simulink subsystem "ros_command"  (R2024a)
settings: Solver=VariableStepAuto  StartTime=0.0  StopTime=10.0  RelTol=1e-3
undefined symbols (not defined in the file): MPC, simulink
libraries: ros2lib x43
settings Model: Creator=lamarre  LastModifiedBy=nimai
settings DebuggingCC: UnconnectedInputMsg=warning  UnconnectedOutputMsg=warning  UnconnectedLineMsg=warning
settings ModelReferenceCC: EnableRefExpFcnMdlSchedulingChecks=on
settings RTWCC: GPUComputeCapability=3.5  DLArmComputeVersion=19.05

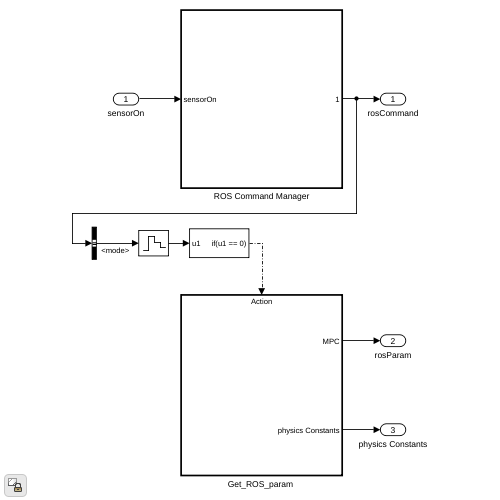
[thumbnail: Simulink's stored preview of the top-level diagram]
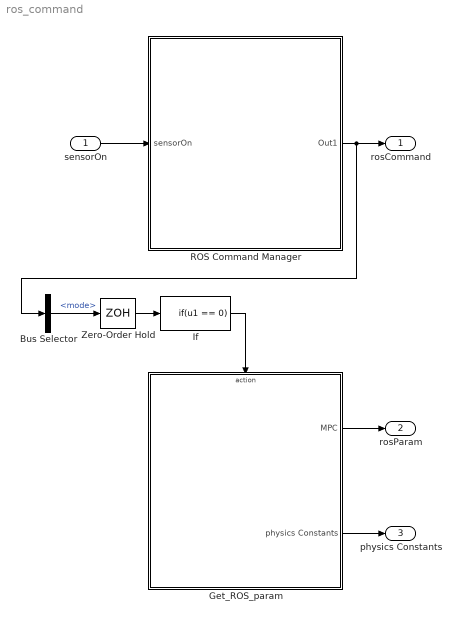
== system ros_command ==
  sensorOn : Inport
  Bus Selector : BusSelector  OutputSignals=mode
  "Get_ROS_param " : Subsystem
  If : If  IfExpression=u1 == 0  ShowElse=off
  ROS Command Manager : Subsystem  TreatAsAtomicUnit=on  SystemSampleTime=MPC.Ts
  Zero-Order Hold : ZeroOrderHold  SampleTime=simulink.ros.paramSampletime
  rosCommand : Outport
  rosParam : Outport  Port=2
  physics Constants : Outport  Port=3
  wires:
  sensorOn/1 -> ROS Command Manager/1(sensorOn)
  ROS Command Manager/1(Out1) -> Bus Selector/1, rosCommand/1
  If/1 -> "Get_ROS_param "/Action
  Bus Selector/1 -> Zero-Order Hold/1  "<mode>"
  "Get_ROS_param "/1(MPC) -> rosParam/1
  "Get_ROS_param "/2(physics Constants) -> physics Constants/1
  Zero-Order Hold/1 -> If/1

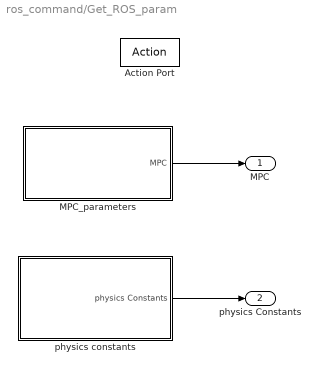
== system ros_command/Get_ROS_param  ==
  Action Port : ActionPort  InitializeStates=reset
  MPC_parameters : Subsystem
  physics constants : Subsystem
  MPC : Outport
  physics Constants : Outport  Port=2
  wires:
  physics constants/1(physics Constants) -> physics Constants/1
  MPC_parameters/1(MPC) -> MPC/1

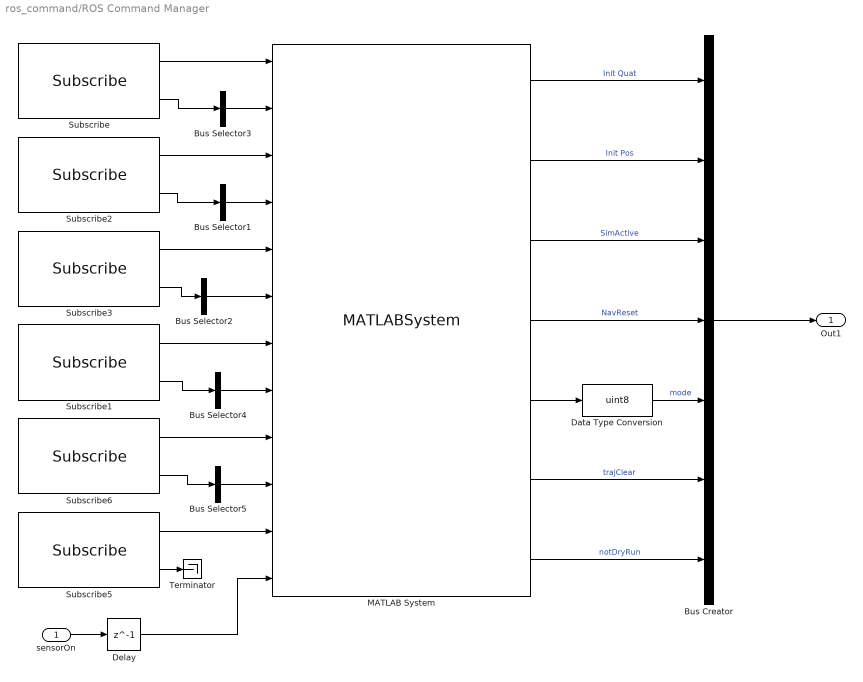
== system ros_command/ROS Command Manager ==
  sensorOn : Inport
  Bus Creator : BusCreator  Inputs=7
  Bus Selector{1..3,5} (4 alike) : BusSelector  OutputSignals=Data  OutputAsBus=on
  Bus Selector4 : BusSelector  OutputSignals=Position.X,Position.Y,Position.Z,Orientation.W,Orientation.X,Orientation.Y,Orientation.Z  OutputAsBus=on
  Data Type Conversion : DataTypeConversion  OutDataTypeStr=uint8  SaturateOnIntegerOverflow=off  RndMeth=Floor
  Delay : Delay  DelayLength=1  InitialCondition=0
  MATLAB System : MATLABSystem  System=rosCommandManager  initial_mode=mode.init  SimulateUsing=Code generation
      mask Type: rosCommandManager
      mask Display:
      | disp('rosCommandManager');
      | port_label('input',1,'newSetMode');
      | port_label('input',2,'setMode');
      | port_label('input',3,'newReset');
      | port_label('input',4,'reset');
      | port_label('input',5,'newKill');
      | port_label('input',6,'kill');
      | port_label('input',7,'newIc');
      | port_label('input',8,'ic');
      | port_label('input',9,'newDryRun');
      | port_label('input',10,'Dryrun');
      | port_label('input',11,'newTrajreset');
      | port_label('input',12,'sensorOn');
      | port_label('output',1,'initQuat');
      | port_label('output',2,'initPos');
      | port_label('output',3,'simEnable');
      | port_label('output',4,'reset');
      | port_label('output',5,'mode');
      | port_label('output',6,'trajClear');
      | port_label('output',7,'notDryRun');
  Subscribe : ros2lib/Subscribe  topicSource=Specify your own  topic=/proc_control/set_mode  messageType=std_msgs/UInt8  sampleTime=MPC.Ts  QOSHistory=Keep last  QOSDepth=1  QOSReliability=Reliable  QOSDurability=Volatile  QOSDeadline=Inf  QOSLifespan=Inf  QOSLiveliness=Automatic  QOSLeaseDuration=Inf  QOSAvoidROSNamespaceConventions=off
  Subscribe1 : ros2lib/Subscribe  topicSource=Specify your own  topic=/proc_simulation/start_simulation  messageType=geometry_msgs/Pose  sampleTime=MPC.Ts  QOSHistory=Keep last  QOSDepth=1  QOSReliability=Reliable  QOSDurability=Volatile  QOSDeadline=Inf  QOSLifespan=Inf  QOSLiveliness=Automatic  QOSLeaseDuration=Inf  QOSAvoidROSNamespaceConventions=off
  Subscribe2 : ros2lib/Subscribe  topicSource=Specify your own  topic=/proc_nav/reset_pos  messageType=std_msgs/Bool  sampleTime=MPC.Ts  QOSHistory=Keep last  QOSDepth=1  QOSReliability=Reliable  QOSDurability=Volatile  QOSDeadline=Inf  QOSLifespan=Inf  QOSLiveliness=Automatic  QOSLeaseDuration=Inf  QOSAvoidROSNamespaceConventions=off
  Subscribe3 : ros2lib/Subscribe  topicSource=Specify your own  topic=/provider_rs485/kill_status  messageType=sonia_common_ros2/KillStatus  sampleTime=MPC.Ts  QOSHistory=Keep last  QOSDepth=1  QOSReliability=Reliable  QOSDurability=Volatile  QOSDeadline=Inf  QOSLifespan=Inf  QOSLiveliness=Automatic  QOSLeaseDuration=Inf  QOSAvoidROSNamespaceConventions=off
  Subscribe5 : ros2lib/Subscribe  topicSource=Specify your own  topic=/proc_control/reset_trajectory  messageType=std_msgs/Bool  sampleTime=MPC.Ts  QOSHistory=Keep last  QOSDepth=1  QOSReliability=Reliable  QOSDurability=Volatile  QOSDeadline=Inf  QOSLifespan=Inf  QOSLiveliness=Automatic  QOSLeaseDuration=Inf  QOSAvoidROSNamespaceConventions=off
  Subscribe6 : ros2lib/Subscribe  topicSource=Specify your own  topic=/telemetry/dry_run  messageType=std_msgs/Bool  sampleTime=MPC.Ts  QOSHistory=Keep last  QOSDepth=1  QOSReliability=Reliable  QOSDurability=Volatile  QOSDeadline=Inf  QOSLifespan=Inf  QOSLiveliness=Automatic  QOSLeaseDuration=Inf  QOSAvoidROSNamespaceConventions=off
  Terminator : Terminator
  Out1 : Outport
  wires:
  Subscribe2/1 -> MATLAB System/3
  Bus Selector5/1 -> MATLAB System/10
  Subscribe1/2 -> Bus Selector4/1
  Subscribe/1 -> MATLAB System/1
  MATLAB System/4 -> Bus Creator/4  "NavReset"
  Subscribe5/1 -> MATLAB System/11
  Bus Selector2/1 -> MATLAB System/6
  Bus Creator/1 -> Out1/1
  Bus Selector4/1 -> MATLAB System/8
  Subscribe2/2 -> Bus Selector1/1
  MATLAB System/7 -> Bus Creator/7  "notDryRun"
  Data Type Conversion/1 -> Bus Creator/5  "mode"
  sensorOn/1 -> Delay/1
  Subscribe5/2 -> Terminator/1
  Bus Selector3/1 -> MATLAB System/2
  Subscribe1/1 -> MATLAB System/7
  MATLAB System/3 -> Bus Creator/3  "SimActive"
  Subscribe6/2 -> Bus Selector5/1
  Subscribe3/1 -> MATLAB System/5
  Subscribe/2 -> Bus Selector3/1
  Subscribe3/2 -> Bus Selector2/1
  Bus Selector1/1 -> MATLAB System/4
  Delay/1 -> MATLAB System/12
  Subscribe6/1 -> MATLAB System/9
  MATLAB System/6 -> Bus Creator/6  "trajClear"
  MATLAB System/2 -> Bus Creator/2  "Init Pos"
  MATLAB System/5 -> Data Type Conversion/1
  MATLAB System/1 -> Bus Creator/1  "Init Quat"

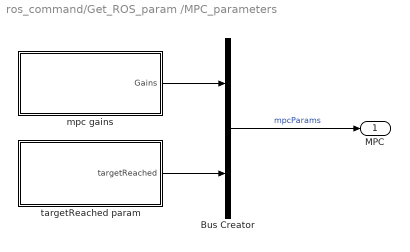
== system ros_command/Get_ROS_param /MPC_parameters ==
  Bus Creator : BusCreator  Inputs=2  OutDataTypeStr=Bus: mpcParams  NonVirtualBus=on
  mpc gains : Subsystem
  targetReached param : Subsystem
  MPC : Outport
  wires:
  Bus Creator/1 -> MPC/1  "mpcParams"
  mpc gains/1(Gains) -> Bus Creator/1
  targetReached param/1(targetReached) -> Bus Creator/2

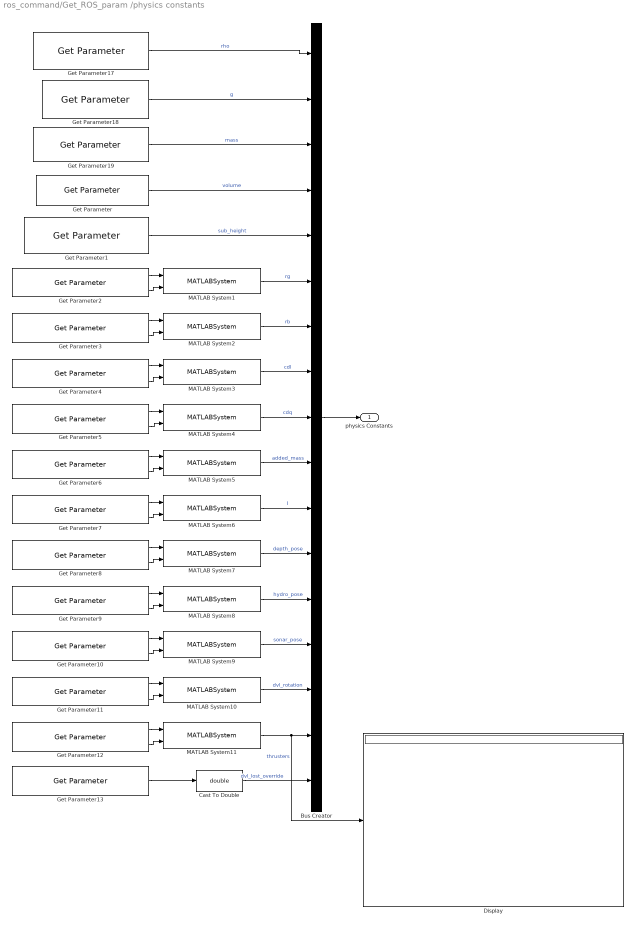
== system ros_command/Get_ROS_param /physics constants ==
  Bus Creator : BusCreator  Inputs=17  OutDataTypeStr=Bus: physicsConstants  NonVirtualBus=on
  Cast To Double : DataTypeConversion  OutDataTypeStr=double  SaturateOnIntegerOverflow=off  RndMeth=Floor
  Display : Display
  Get Parameter : ros2lib/Get Parameter  ParameterName=proc_control.physics.volume  ParameterType=double  ParameterMaxArrayLength=16  ParameterInitialValue=physics.volume  SampleTime=-1  ModelName=proc_control  BlockId=ParamGet_proc_control_185_615
  Get Parameter1 : ros2lib/Get Parameter  ParameterName=proc_control.physics.sub_height  ParameterType=double  ParameterMaxArrayLength=16  ParameterInitialValue=physics.height  SampleTime=-1  ModelName=proc_control  BlockId=ParamGet_proc_control_185_616
  Get Parameter10 : ros2lib/Get Parameter  ParameterName=proc_control.physics.sonar_pose  ParameterType=uint8[]  ParameterMaxArrayLength=64  ParameterInitialValue=int8('0,0,0')  SampleTime=-1  ModelName=proc_control  BlockId=ParamGet_proc_control_185_626
  Get Parameter11 : ros2lib/Get Parameter  ParameterName=proc_control.physics.dvl_rotation  ParameterType=uint8[]  ParameterMaxArrayLength=64  ParameterInitialValue=int8('0,0,0')  SampleTime=-1  ModelName=proc_control  BlockId=ParamGet_proc_control_185_627
  Get Parameter12 : ros2lib/Get Parameter  ParameterName=proc_control.physics.thrusters  ParameterType=uint8[]  ParameterMaxArrayLength=400  ParameterInitialValue=int8('0,0,0')  SampleTime=-1  ModelName=proc_control  BlockId=ParamGet_proc_control_185_628
  Get Parameter13 : ros2lib/Get Parameter  ParameterName=proc_control.physics.dvl_lost_override  ParameterType=boolean  ParameterMaxArrayLength=400  ParameterInitialValue=true  SampleTime=-1  ModelName=proc_control  BlockId=ParamGet_proc_control_185_629
  Get Parameter17 : ros2lib/Get Parameter  ParameterName=proc_control.physics.rho  ParameterType=double  ParameterMaxArrayLength=16  ParameterInitialValue=physics.rho  SampleTime=-1  ModelName=proc_control  BlockId=ParamGet_proc_control_185_612
  Get Parameter18 : ros2lib/Get Parameter  ParameterName=proc_control.physics.g  ParameterType=double  ParameterMaxArrayLength=16  ParameterInitialValue=physics.g  SampleTime=-1  ModelName=proc_control  BlockId=ParamGet_proc_control_185_613
  Get Parameter19 : ros2lib/Get Parameter  ParameterName=proc_control.physics.mass  ParameterType=double  ParameterMaxArrayLength=16  ParameterInitialValue=physics.mass  SampleTime=-1  ModelName=proc_control  BlockId=ParamGet_proc_control_185_614
  Get Parameter2 : ros2lib/Get Parameter  ParameterName=proc_control.physics.rg  ParameterType=uint8[]  ParameterMaxArrayLength=64  ParameterInitialValue=int8('0,0,0')  SampleTime=-1  ModelName=proc_control  BlockId=ParamGet_proc_control_185_617
  Get Parameter3 : ros2lib/Get Parameter  ParameterName=proc_control.physics.rb  ParameterType=uint8[]  ParameterMaxArrayLength=64  ParameterInitialValue=int8('0,0,0')  SampleTime=-1  ModelName=proc_control  BlockId=ParamGet_proc_control_185_618
  Get Parameter4 : ros2lib/Get Parameter  ParameterName=proc_control.physics.cdl  ParameterType=uint8[]  ParameterMaxArrayLength=64  ParameterInitialValue=int8('0,0,0,0,0,0')  SampleTime=-1  ModelName=proc_control  BlockId=ParamGet_proc_control_185_619
  Get Parameter5 : ros2lib/Get Parameter  ParameterName=proc_control.physics.cdq  ParameterType=uint8[]  ParameterMaxArrayLength=64  ParameterInitialValue=int8('0,0,0,0,0,0')  SampleTime=-1  ModelName=proc_control  BlockId=ParamGet_proc_control_185_620
  Get Parameter6 : ros2lib/Get Parameter  ParameterName=proc_control.physics.added_mass  ParameterType=uint8[]  ParameterMaxArrayLength=64  ParameterInitialValue=int8('0,0,0,0,0,0')  SampleTime=-1  ModelName=proc_control  BlockId=ParamGet_proc_control_185_621
  Get Parameter7 : ros2lib/Get Parameter  ParameterName=proc_control.physics.I  ParameterType=uint8[]  ParameterMaxArrayLength=128  ParameterInitialValue=int8('0,0,0,0,0,0,0,0,0')  SampleTime=-1  ModelName=proc_control  BlockId=ParamGet_proc_control_185_622
  Get Parameter8 : ros2lib/Get Parameter  ParameterName=proc_control.physics.depth_pose  ParameterType=uint8[]  ParameterMaxArrayLength=64  ParameterInitialValue=int8('0,0,0')  SampleTime=-1  ModelName=proc_control  BlockId=ParamGet_proc_control_185_623
  Get Parameter9 : ros2lib/Get Parameter  ParameterName=proc_control.physics.hydro_pose  ParameterType=uint8[]  ParameterMaxArrayLength=64  ParameterInitialValue=int8('0,0,0')  SampleTime=-1  ModelName=proc_control  BlockId=ParamGet_proc_control_185_625
  MATLAB System1 : MATLABSystem  System=String2DoubleArray  arraySize=[1, 3]  constantName='Center of Mass'  SimulateUsing=Code generation
      mask Type: String2DoubleArray
      mask Display:
      | disp('String2DoubleArray');
      | port_label('input',1,'string');
      | port_label('input',2,'length');
      | port_label('output',1,'array');
  MATLAB System10 : MATLABSystem  System=String2DoubleArray  arraySize=[1, 3]  constantName='DVL Rotation'  SimulateUsing=Code generation
      mask Type: String2DoubleArray
      mask Display:
      | disp('String2DoubleArray');
      | port_label('input',1,'string');
      | port_label('input',2,'length');
      | port_label('output',1,'array');
  MATLAB System11 : MATLABSystem  System=String2DoubleArray  arraySize=[MPC.nu 6]  constantName='Thrusters Config'  SimulateUsing=Code generation
      mask Type: String2DoubleArray
      mask Display:
      | disp('String2DoubleArray');
      | port_label('input',1,'string');
      | port_label('input',2,'length');
      | port_label('output',1,'array');
  MATLAB System2 : MATLABSystem  System=String2DoubleArray  arraySize=[1, 3]  constantName='Center of Buoyancy'  SimulateUsing=Code generation
      mask Type: String2DoubleArray
      mask Display:
      | disp('String2DoubleArray');
      | port_label('input',1,'string');
      | port_label('input',2,'length');
      | port_label('output',1,'array');
  MATLAB System3 : MATLABSystem  System=String2DoubleArray  arraySize=[1,6]  constantName='Linear drag constant'  SimulateUsing=Code generation
      mask Type: String2DoubleArray
      mask Display:
      | disp('String2DoubleArray');
      | port_label('input',1,'string');
      | port_label('input',2,'length');
      | port_label('output',1,'array');
  MATLAB System4 : MATLABSystem  System=String2DoubleArray  arraySize=[1, 6]  constantName='Quadratic drag constant'  SimulateUsing=Code generation
      mask Type: String2DoubleArray
      mask Display:
      | disp('String2DoubleArray');
      | port_label('input',1,'string');
      | port_label('input',2,'length');
      | port_label('output',1,'array');
  MATLAB System5 : MATLABSystem  System=String2DoubleArray  arraySize=[1, 6]  constantName='Added Mass'  SimulateUsing=Code generation
      mask Type: String2DoubleArray
      mask Display:
      | disp('String2DoubleArray');
      | port_label('input',1,'string');
      | port_label('input',2,'length');
      | port_label('output',1,'array');
  MATLAB System6 : MATLABSystem  System=String2DoubleArray  arraySize=[1,9]  constantName='Inertia Tensor'  SimulateUsing=Code generation
      mask Type: String2DoubleArray
      mask Display:
      | disp('String2DoubleArray');
      | port_label('input',1,'string');
      | port_label('input',2,'length');
      | port_label('output',1,'array');
  MATLAB System7 : MATLABSystem  System=String2DoubleArray  arraySize=[1, 3]  constantName='Depth Pose'  SimulateUsing=Code generation
      mask Type: String2DoubleArray
      mask Display:
      | disp('String2DoubleArray');
      | port_label('input',1,'string');
      | port_label('input',2,'length');
      | port_label('output',1,'array');
  MATLAB System8 : MATLABSystem  System=String2DoubleArray  arraySize=[1, 3]  constantName='Hydro Pose'  SimulateUsing=Code generation
      mask Type: String2DoubleArray
      mask Display:
      | disp('String2DoubleArray');
      | port_label('input',1,'string');
      | port_label('input',2,'length');
      | port_label('output',1,'array');
  MATLAB System9 : MATLABSystem  System=String2DoubleArray  arraySize=[1, 3]  constantName='Sonar Pose'  SimulateUsing=Code generation
      mask Type: String2DoubleArray
      mask Display:
      | disp('String2DoubleArray');
      | port_label('input',1,'string');
      | port_label('input',2,'length');
      | port_label('output',1,'array');
  physics Constants : Outport
  wires:
  Cast To Double/1 -> Bus Creator/17  "dvl_lost_override"
  Get Parameter13/1 -> Cast To Double/1
  MATLAB System11/1 -> Bus Creator/16, Display/1  "thrusters"
  Get Parameter12/2 -> MATLAB System11/2
  Get Parameter12/1 -> MATLAB System11/1
  MATLAB System10/1 -> Bus Creator/15  "dvl_rotation"
  Get Parameter11/1 -> MATLAB System10/1
  Get Parameter11/2 -> MATLAB System10/2
  MATLAB System9/1 -> Bus Creator/14  "sonar_pose"
  Get Parameter10/1 -> MATLAB System9/1
  Get Parameter10/2 -> MATLAB System9/2
  MATLAB System8/1 -> Bus Creator/13  "hydro_pose"
  Get Parameter9/1 -> MATLAB System8/1
  Get Parameter9/2 -> MATLAB System8/2
  MATLAB System7/1 -> Bus Creator/12  "depth_pose"
  Get Parameter8/2 -> MATLAB System7/2
  Get Parameter8/1 -> MATLAB System7/1
  MATLAB System6/1 -> Bus Creator/11  "I"
  Get Parameter7/1 -> MATLAB System6/1
  Get Parameter7/2 -> MATLAB System6/2
  MATLAB System5/1 -> Bus Creator/10  "added_mass"
  Get Parameter6/1 -> MATLAB System5/1
  Get Parameter6/2 -> MATLAB System5/2
  MATLAB System4/1 -> Bus Creator/9  "cdq"
  MATLAB System3/1 -> Bus Creator/8  "cdl"
  Get Parameter5/2 -> MATLAB System4/2
  Get Parameter4/2 -> MATLAB System3/2
  Get Parameter4/1 -> MATLAB System3/1
  Get Parameter5/1 -> MATLAB System4/1
  MATLAB System2/1 -> Bus Creator/7  "rb"
  Get Parameter3/2 -> MATLAB System2/2
  Get Parameter3/1 -> MATLAB System2/1
  MATLAB System1/1 -> Bus Creator/6  "rg"
  Get Parameter2/2 -> MATLAB System1/2
  Get Parameter2/1 -> MATLAB System1/1
  Get Parameter1/1 -> Bus Creator/5  "sub_height"
  Get Parameter/1 -> Bus Creator/4  "volume"
  Get Parameter19/1 -> Bus Creator/3  "mass"
  Get Parameter18/1 -> Bus Creator/2  "g"
  Bus Creator/1 -> physics Constants/1
  Get Parameter17/1 -> Bus Creator/1  "rho"

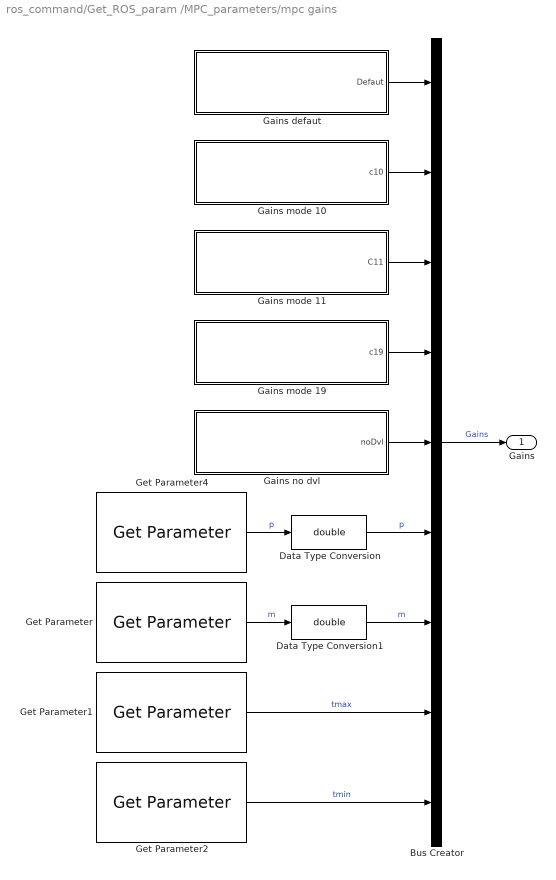
== system ros_command/Get_ROS_param /MPC_parameters/mpc gains ==
  Bus Creator : BusCreator  Inputs=9
  Data Type Conversion : DataTypeConversion  OutDataTypeStr=double  SaturateOnIntegerOverflow=off  RndMeth=Floor
  Data Type Conversion1 : DataTypeConversion  OutDataTypeStr=double  SaturateOnIntegerOverflow=off  RndMeth=Floor
  Gains defaut : Subsystem
  Gains mode 10 : Subsystem
  Gains mode 11 : Subsystem
  Gains mode 19 : Subsystem
  Gains no dvl : Subsystem
  Get Parameter : ros2lib/Get Parameter  ParameterName=proc_control.mpc.m  ParameterType=int64  ParameterMaxArrayLength=16  ParameterInitialValue=MPC.m  SampleTime=-1  ModelName=proc_control  BlockId=ParamGet_proc_control_185_593
  Get Parameter1 : ros2lib/Get Parameter  ParameterName=proc_control.mpc.tmax  ParameterType=double  ParameterMaxArrayLength=16  ParameterInitialValue=MPC.tmax  SampleTime=-1  ModelName=proc_control  BlockId=ParamGet_proc_control_185_594
  Get Parameter2 : ros2lib/Get Parameter  ParameterName=proc_control.mpc.tmin  ParameterType=double  ParameterMaxArrayLength=16  ParameterInitialValue=MPC.tmin  SampleTime=-1  ModelName=proc_control  BlockId=ParamGet_proc_control_185_595
  Get Parameter4 : ros2lib/Get Parameter  ParameterName=proc_control.mpc.p  ParameterType=int64  ParameterMaxArrayLength=16  ParameterInitialValue=MPC.p  SampleTime=-1  ModelName=proc_control  BlockId=ParamGet_proc_control_185_592
  Gains : Outport
  wires:
  Get Parameter2/1 -> Bus Creator/9  "tmin"
  Get Parameter1/1 -> Bus Creator/8  "tmax"
  Get Parameter/1 -> Data Type Conversion1/1  "m"
  Get Parameter4/1 -> Data Type Conversion/1  "p"
  Data Type Conversion1/1 -> Bus Creator/7  "m"
  Data Type Conversion/1 -> Bus Creator/6  "p"
  Gains no dvl/1(noDvl) -> Bus Creator/5
  Gains defaut/1(Defaut) -> Bus Creator/1
  Gains mode 10/1(c10) -> Bus Creator/2
  Bus Creator/1 -> Gains/1  "Gains"
  Gains mode 19/1(c19) -> Bus Creator/4
  Gains mode 11/1(C11) -> Bus Creator/3

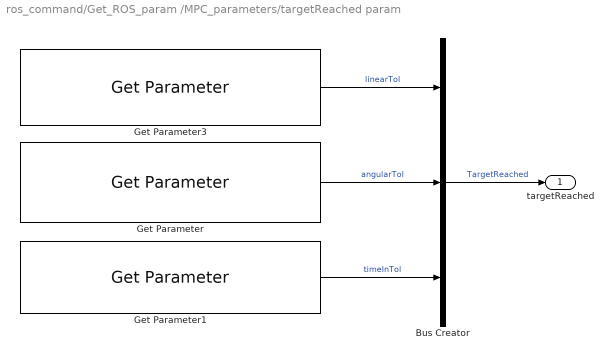
== system ros_command/Get_ROS_param /MPC_parameters/targetReached param ==
  Bus Creator : BusCreator  Inputs=3
  Get Parameter : ros2lib/Get Parameter  ParameterName=proc_control.target_reached.angular_tolerance  ParameterType=double  ParameterMaxArrayLength=16  ParameterInitialValue=MPC.targetReached.angularTol  SampleTime=-1  ModelName=proc_control  BlockId=ParamGet_proc_control_185_610
  Get Parameter1 : ros2lib/Get Parameter  ParameterName=proc_control.target_reached.time_in_tolerance  ParameterType=double  ParameterMaxArrayLength=16  ParameterInitialValue=MPC.targetReached.timeInTol  SampleTime=-1  ModelName=proc_control  BlockId=ParamGet_proc_control_185_611
  Get Parameter3 : ros2lib/Get Parameter  ParameterName=proc_control.target_reached.linear_tolerance  ParameterType=double  ParameterMaxArrayLength=16  ParameterInitialValue=MPC.targetReached.linearTol  SampleTime=-1  ModelName=proc_control  BlockId=ParamGet_proc_control_185_609
  targetReached : Outport
  wires:
  Bus Creator/1 -> targetReached/1  "TargetReached"
  Get Parameter/1 -> Bus Creator/2  "angularTol"
  Get Parameter3/1 -> Bus Creator/1  "linearTol"
  Get Parameter1/1 -> Bus Creator/3  "timeInTol"

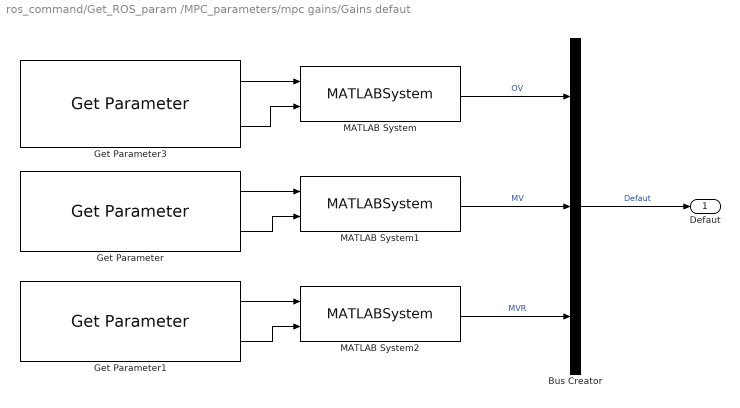
== system ros_command/Get_ROS_param /MPC_parameters/mpc gains/Gains defaut ==
  Bus Creator : BusCreator  Inputs=3
  Get Parameter : ros2lib/Get Parameter  ParameterName=proc_control.mpc.gains.default.mv  ParameterType=uint8[]  ParameterMaxArrayLength=64  ParameterInitialValue=uint8('30,30,30,45,45,45,45,0,0,0,0,0,0')  SampleTime=-1  ModelName=proc_control  BlockId=ParamGet_proc_control_185_597
  Get Parameter1 : ros2lib/Get Parameter  ParameterName=proc_control.mpc.gains.default.mvr  ParameterType=uint8[]  ParameterMaxArrayLength=64  ParameterInitialValue=uint8('30,30,30,45,45,45,45,0,0,0,0,0,0')  SampleTime=-1  ModelName=proc_control  BlockId=ParamGet_proc_control_185_598
  Get Parameter3 : ros2lib/Get Parameter  ParameterName=proc_control.mpc.gains.default.ov  ParameterType=uint8[]  ParameterMaxArrayLength=64  ParameterInitialValue=uint8('30,30,30,45,45,45,45,0,0,0,0,0,0')  SampleTime=-1  ModelName=proc_control  BlockId=ParamGet_proc_control_185_596
  MATLAB System : MATLABSystem  System=String2DoubleArray  arraySize=[1 MPC.nx]  constantName='Default OV'  SimulateUsing=Code generation
      mask Type: String2DoubleArray
      mask Display:
      | disp('String2DoubleArray');
      | port_label('input',1,'string');
      | port_label('input',2,'length');
      | port_label('output',1,'array');
  MATLAB System1 : MATLABSystem  System=String2DoubleArray  arraySize=[1 MPC.nu]  constantName='Default MV'  SimulateUsing=Code generation
      mask Type: String2DoubleArray
      mask Display:
      | disp('String2DoubleArray');
      | port_label('input',1,'string');
      | port_label('input',2,'length');
      | port_label('output',1,'array');
  MATLAB System2 : MATLABSystem  System=String2DoubleArray  arraySize=[1 MPC.nu]  constantName='Default MVR'  SimulateUsing=Code generation
      mask Type: String2DoubleArray
      mask Display:
      | disp('String2DoubleArray');
      | port_label('input',1,'string');
      | port_label('input',2,'length');
      | port_label('output',1,'array');
  Defaut : Outport
  wires:
  MATLAB System2/1 -> Bus Creator/3  "MVR"
  MATLAB System/1 -> Bus Creator/1  "OV"
  Get Parameter3/1 -> MATLAB System/1
  Bus Creator/1 -> Defaut/1  "Defaut"
  Get Parameter/1 -> MATLAB System1/1
  Get Parameter1/2 -> MATLAB System2/2
  MATLAB System1/1 -> Bus Creator/2  "MV"
  Get Parameter/2 -> MATLAB System1/2
  Get Parameter3/2 -> MATLAB System/2
  Get Parameter1/1 -> MATLAB System2/1

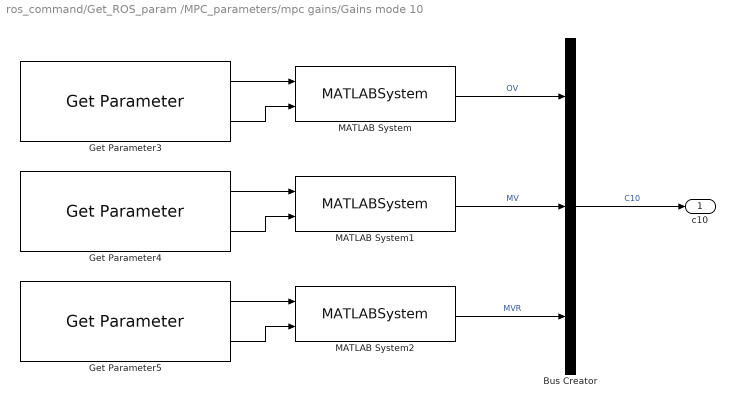
== system ros_command/Get_ROS_param /MPC_parameters/mpc gains/Gains mode 10 ==
  Bus Creator : BusCreator  Inputs=3
  Get Parameter3 : ros2lib/Get Parameter  ParameterName=proc_control.mpc.gains.c10.ov  ParameterType=uint8[]  ParameterMaxArrayLength=64  ParameterInitialValue=uint8('30,30,30,45,45,45,45,0,0,0,0,0,0')  SampleTime=-1  ModelName=proc_control  BlockId=ParamGet_proc_control_185_599
  Get Parameter4 : ros2lib/Get Parameter  ParameterName=proc_control.mpc.gains.c10.mv  ParameterType=uint8[]  ParameterMaxArrayLength=64  ParameterInitialValue=uint8('30,30,30,45,45,45,45,0,0,0,0,0,0')  SampleTime=-1  ModelName=proc_control  BlockId=ParamGet_proc_control_185_600
  Get Parameter5 : ros2lib/Get Parameter  ParameterName=proc_control.mpc.gains.c10.mvr  ParameterType=uint8[]  ParameterMaxArrayLength=64  ParameterInitialValue=uint8('30,30,30,45,45,45,45,0,0,0,0,0,0')  SampleTime=-1  ModelName=proc_control  BlockId=ParamGet_proc_control_185_601
  MATLAB System : MATLABSystem  System=String2DoubleArray  arraySize=[1 MPC.nx]  constantName='M10 OV'  SimulateUsing=Code generation
      mask Type: String2DoubleArray
      mask Display:
      | disp('String2DoubleArray');
      | port_label('input',1,'string');
      | port_label('input',2,'length');
      | port_label('output',1,'array');
  MATLAB System1 : MATLABSystem  System=String2DoubleArray  arraySize=[1 MPC.nu]  constantName='M10 MV'  SimulateUsing=Code generation
      mask Type: String2DoubleArray
      mask Display:
      | disp('String2DoubleArray');
      | port_label('input',1,'string');
      | port_label('input',2,'length');
      | port_label('output',1,'array');
  MATLAB System2 : MATLABSystem  System=String2DoubleArray  arraySize=[1 MPC.nu]  constantName='M10 MVR'  SimulateUsing=Code generation
      mask Type: String2DoubleArray
      mask Display:
      | disp('String2DoubleArray');
      | port_label('input',1,'string');
      | port_label('input',2,'length');
      | port_label('output',1,'array');
  c10 : Outport
  wires:
  MATLAB System2/1 -> Bus Creator/3  "MVR"
  MATLAB System/1 -> Bus Creator/1  "OV"
  Get Parameter3/1 -> MATLAB System/1
  Bus Creator/1 -> c10/1  "C10"
  Get Parameter4/1 -> MATLAB System1/1
  Get Parameter5/2 -> MATLAB System2/2
  MATLAB System1/1 -> Bus Creator/2  "MV"
  Get Parameter4/2 -> MATLAB System1/2
  Get Parameter3/2 -> MATLAB System/2
  Get Parameter5/1 -> MATLAB System2/1

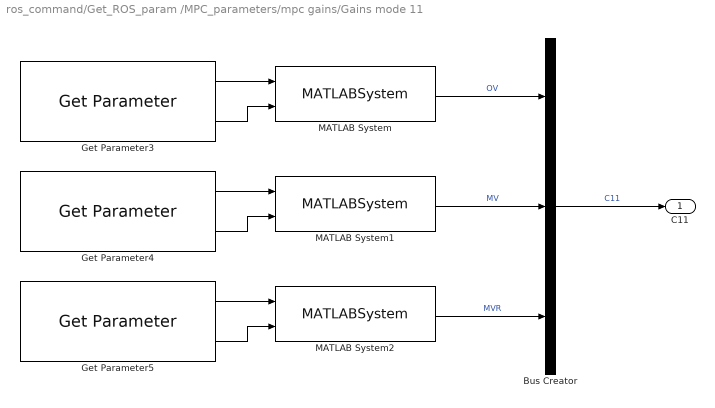
== system ros_command/Get_ROS_param /MPC_parameters/mpc gains/Gains mode 11 ==
  Bus Creator : BusCreator  Inputs=3
  Get Parameter3 : ros2lib/Get Parameter  ParameterName=proc_control.mpc.gains.c11.ov  ParameterType=uint8[]  ParameterMaxArrayLength=64  ParameterInitialValue=uint8('30,30,30,45,45,45,45,0,0,0,0,0,0')  SampleTime=-1  ModelName=proc_control  BlockId=ParamGet_proc_control_185_602
  Get Parameter4 : ros2lib/Get Parameter  ParameterName=proc_control.mpc.gains.c11.mv  ParameterType=uint8[]  ParameterMaxArrayLength=64  ParameterInitialValue=uint8('30,30,30,45,45,45,45,0,0,0,0,0,0')  SampleTime=-1  ModelName=proc_control  BlockId=ParamGet_proc_control_185_603
  Get Parameter5 : ros2lib/Get Parameter  ParameterName=proc_control.mpc.gains.c11.mvr  ParameterType=uint8[]  ParameterMaxArrayLength=64  ParameterInitialValue=uint8('30,30,30,45,45,45,45,0,0,0,0,0,0')  SampleTime=-1  ModelName=proc_control  BlockId=ParamGet_proc_control_185_604
  MATLAB System : MATLABSystem  System=String2DoubleArray  arraySize=[1 MPC.nx]  constantName='M11 OV'  SimulateUsing=Code generation
      mask Type: String2DoubleArray
      mask Display:
      | disp('String2DoubleArray');
      | port_label('input',1,'string');
      | port_label('input',2,'length');
      | port_label('output',1,'array');
  MATLAB System1 : MATLABSystem  System=String2DoubleArray  arraySize=[1 MPC.nu]  constantName='M11 MV'  SimulateUsing=Code generation
      mask Type: String2DoubleArray
      mask Display:
      | disp('String2DoubleArray');
      | port_label('input',1,'string');
      | port_label('input',2,'length');
      | port_label('output',1,'array');
  MATLAB System2 : MATLABSystem  System=String2DoubleArray  arraySize=[1 MPC.nu]  constantName='M11 MVR'  SimulateUsing=Code generation
      mask Type: String2DoubleArray
      mask Display:
      | disp('String2DoubleArray');
      | port_label('input',1,'string');
      | port_label('input',2,'length');
      | port_label('output',1,'array');
  C11 : Outport
  wires:
  MATLAB System2/1 -> Bus Creator/3  "MVR"
  MATLAB System/1 -> Bus Creator/1  "OV"
  Get Parameter3/1 -> MATLAB System/1
  Bus Creator/1 -> C11/1  "C11"
  Get Parameter4/1 -> MATLAB System1/1
  Get Parameter5/2 -> MATLAB System2/2
  MATLAB System1/1 -> Bus Creator/2  "MV"
  Get Parameter4/2 -> MATLAB System1/2
  Get Parameter3/2 -> MATLAB System/2
  Get Parameter5/1 -> MATLAB System2/1

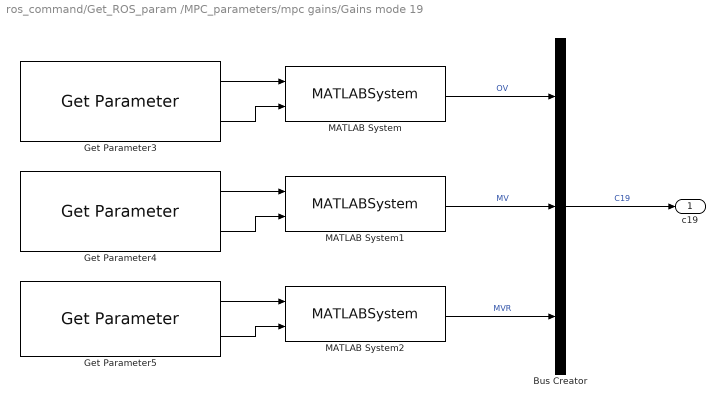
== system ros_command/Get_ROS_param /MPC_parameters/mpc gains/Gains mode 19 ==
  Bus Creator : BusCreator  Inputs=3
  Get Parameter3 : ros2lib/Get Parameter  ParameterName=proc_control.mpc.gains.c19.ov  ParameterType=uint8[]  ParameterMaxArrayLength=64  ParameterInitialValue=uint8('30,30,30,45,45,45,45,0,0,0,0,0,0')  SampleTime=-1  ModelName=proc_control  BlockId=ParamGet_proc_control_185_605
  Get Parameter4 : ros2lib/Get Parameter  ParameterName=proc_control.mpc.gains.c19.mv  ParameterType=uint8[]  ParameterMaxArrayLength=64  ParameterInitialValue=uint8('30,30,30,45,45,45,45,0,0,0,0,0,0')  SampleTime=-1  ModelName=proc_control  BlockId=ParamGet_proc_control_185_606
  Get Parameter5 : ros2lib/Get Parameter  ParameterName=proc_control.mpc.gains.c19.mvr  ParameterType=uint8[]  ParameterMaxArrayLength=64  ParameterInitialValue=uint8('30,30,30,45,45,45,45,0,0,0,0,0,0')  SampleTime=-1  ModelName=proc_control  BlockId=ParamGet_proc_control_185_607
  MATLAB System : MATLABSystem  System=String2DoubleArray  arraySize=[1 MPC.nx]  constantName='M19 OV'  SimulateUsing=Code generation
      mask Type: String2DoubleArray
      mask Display:
      | disp('String2DoubleArray');
      | port_label('input',1,'string');
      | port_label('input',2,'length');
      | port_label('output',1,'array');
  MATLAB System1 : MATLABSystem  System=String2DoubleArray  arraySize=[1 MPC.nu]  constantName='M19 MV'  SimulateUsing=Code generation
      mask Type: String2DoubleArray
      mask Display:
      | disp('String2DoubleArray');
      | port_label('input',1,'string');
      | port_label('input',2,'length');
      | port_label('output',1,'array');
  MATLAB System2 : MATLABSystem  System=String2DoubleArray  arraySize=[1 MPC.nu]  constantName='M19 MVR'  SimulateUsing=Code generation
      mask Type: String2DoubleArray
      mask Display:
      | disp('String2DoubleArray');
      | port_label('input',1,'string');
      | port_label('input',2,'length');
      | port_label('output',1,'array');
  c19 : Outport
  wires:
  MATLAB System2/1 -> Bus Creator/3  "MVR"
  MATLAB System/1 -> Bus Creator/1  "OV"
  Get Parameter3/1 -> MATLAB System/1
  Bus Creator/1 -> c19/1  "C19"
  Get Parameter4/1 -> MATLAB System1/1
  Get Parameter5/2 -> MATLAB System2/2
  MATLAB System1/1 -> Bus Creator/2  "MV"
  Get Parameter4/2 -> MATLAB System1/2
  Get Parameter3/2 -> MATLAB System/2
  Get Parameter5/1 -> MATLAB System2/1

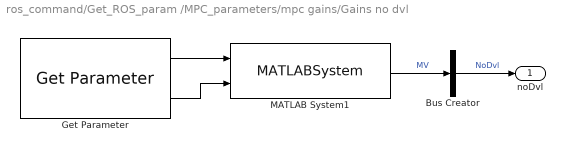
== system ros_command/Get_ROS_param /MPC_parameters/mpc gains/Gains no dvl ==
  Bus Creator : BusCreator  Inputs=1
  Get Parameter : ros2lib/Get Parameter  ParameterName=proc_control.mpc.gains.noDvl.mv  ParameterType=uint8[]  ParameterMaxArrayLength=64  ParameterInitialValue=uint8('30,30,30,45,45,45,45,0,0,0,0,0,0')  SampleTime=-1  ModelName=proc_control  BlockId=ParamGet_proc_control_185_608
  MATLAB System1 : MATLABSystem  System=String2DoubleArray  arraySize=[1 MPC.nu]  constantName='No DVL MV'  SimulateUsing=Code generation
      mask Type: String2DoubleArray
      mask Display:
      | disp('String2DoubleArray');
      | port_label('input',1,'string');
      | port_label('input',2,'length');
      | port_label('output',1,'array');
  noDvl : Outport
  wires:
  MATLAB System1/1 -> Bus Creator/1  "MV"
  Bus Creator/1 -> noDvl/1  "NoDvl"
  Get Parameter/1 -> MATLAB System1/1
  Get Parameter/2 -> MATLAB System1/2
